simulink model "Codegen"  (Simulink 10.2)
settings: Solver=FixedStepDiscrete  StartTime=0.0  StopTime=10.0  FixedStep=dT  RelTol=1e-3  EnableMultiTasking=on
values from neighbouring files (symbols this model uses):
  a1 = mpt.Parameter    [data_object_def.m]
  a2 = mpt.Parameter    [data_object_def.m]
  b1 = mpt.Parameter    [data_object_def.m]
  b2 = mpt.Parameter    [data_object_def.m]
  dT = mpt.Parameter    [data_object_def.m]
  eta = mpt.Parameter    [data_object_def.m]
  Kp = mpt.Parameter    [data_object_def.m]
  Td = mpt.Parameter    [data_object_def.m]
  Ti = mpt.Parameter    [data_object_def.m]
undefined symbols (not defined in the file or in its folder): DiscIntNeverNeededParam
settings Model: Creator=h-mita  LastModifiedBy=yuto
settings DataIOCC: LimitDataPoints=on
settings OptimizationCC: DefaultParameterBehavior=Inlined  ExpressionDepthLimit=2147483647  InitFltsAndDblsToZero=on  LifeSpan=1  EfficientTunableParamExpr=on
settings DebuggingCC: SolverPrmCheckMsg=warning  StateNameClashWarn=warning
settings SFSimCC: SimUseLocalCustomCode=on  MATLABDynamicMemAlloc=off  CustomCodeUndefinedFunction=FilterOut
settings RTWCC: Description=Real-Time Workshop Embedded Coder (no auto configuration)  SystemTargetFile=ert.tlc  GenCodeOnly=on  TemplateMakefile=ert_default_tmf  RTWUseLocalCustomCode=on
settings CodeAppCC: IgnoreCustomStorageClasses=off  CustomSymbolStrType=$N$R$M  InternalIdentifier=Classic
settings ERTTargetCC: GenerateSampleERTMain=on  IncludeMdlTerminateFcn=off  SupportAbsoluteTime=off  SupportComplex=off  InlinedParameterPlacement=NonHierarchical  ERTCustomFileTemplate=example_file_process.tlc  ConvertIfToSwitch=off  SuppressUnreachableDefaultCases=off
settings ConfigComp: CovExternalEMLEnable=on

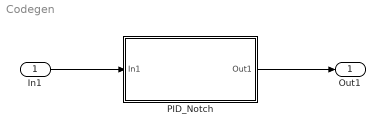
== system Codegen ==
  In1 : Inport
  PID_Notch : Subsystem
  Out1 : Outport  OutDataTypeStr=double
  wires:
  In1/1 -> PID_Notch/1(In1)
  PID_Notch/1(Out1) -> Out1/1

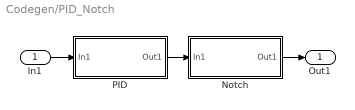
== system Codegen/PID_Notch ==
  In1 : Inport
  Notch : Subsystem
  PID : Subsystem
  Out1 : Outport
  wires:
  PID/1(Out1) -> Notch/1(In1)
  Notch/1(Out1) -> Out1/1
  In1/1 -> PID/1(In1)

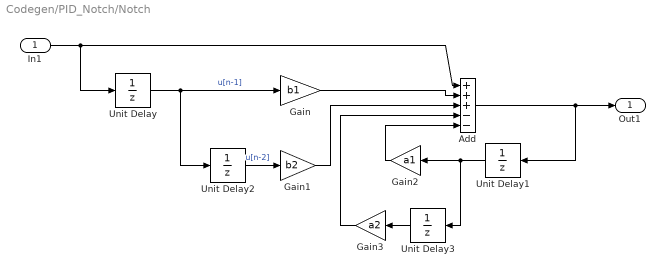
== system Codegen/PID_Notch/Notch ==
  In1 : Inport
  Add : Sum  Inputs=+++--
  Gain : Gain  Gain=b1
  Gain1 : Gain  Gain=b2
  Gain2 : Gain  Gain=a1
  Gain3 : Gain  Gain=a2
  Unit Delay : UnitDelay  SampleTime=-1  StateName=Notch_Unit_Delay  StateMustResolveToSignalObject=on
  Unit Delay1 : UnitDelay  SampleTime=-1  StateName=Notch_Unit_Delay1  StateMustResolveToSignalObject=on
  Unit Delay2 : UnitDelay  SampleTime=-1  StateName=Notch_Unit_Delay2  StateMustResolveToSignalObject=on
  Unit Delay3 : UnitDelay  SampleTime=-1  StateName=Notch_Unit_Delay3  StateMustResolveToSignalObject=on
  Out1 : Outport
  wires:
  Unit Delay/1 -> Gain/1, Unit Delay2/1  "u[n-1]"
  Unit Delay2/1 -> Gain1/1  "u[n-2]"
  Gain1/1 -> Add/3
  Gain/1 -> Add/2
  Add/1 -> Unit Delay1/1, Out1/1
  Unit Delay1/1 -> Gain2/1, Unit Delay3/1
  Gain2/1 -> Add/5
  Unit Delay3/1 -> Gain3/1
  Gain3/1 -> Add/4
  In1/1 -> Unit Delay/1, Add/1

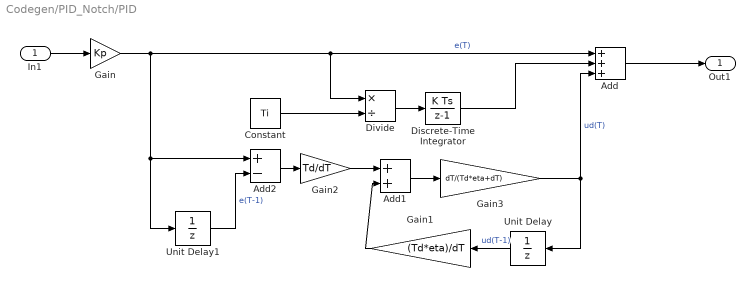
== system Codegen/PID_Notch/PID ==
  In1 : Inport
  Add : Sum  Inputs=+++
  Add1 : Sum
  Add2 : Sum  Inputs=+-
  Constant : Constant  Value=Ti
  Discrete-Time Integrator : DiscreteIntegrator  gainval=1  SampleTime=dT  StateName=PID_Disc_Integrator  ICPrevOutput=DiscIntNeverNeededParam  ICPrevScaledInput=DiscIntNeverNeededParam  StateMustResolveToSignalObject=on
  Divide : Product  Inputs=*/
  Gain : Gain  Gain=Kp
  Gain1 : Gain  Gain=(Td*eta)/dT
  Gain2 : Gain  Gain=Td/dT
  Gain3 : Gain  Gain=dT/(Td*eta+dT)
  Unit Delay : UnitDelay  SampleTime=-1  StateName=PID_Unit_Delay  StateMustResolveToSignalObject=on
  Unit Delay1 : UnitDelay  SampleTime=-1  StateName=PID_Unit_Delay1  StateMustResolveToSignalObject=on
  Out1 : Outport
  wires:
  Gain/1 -> Add/1, Divide/1, Add2/1, Unit Delay1/1  "e(T)"
  Discrete-Time Integrator/1 -> Add/2
  Gain3/1 -> Unit Delay/1, Add/3  "ud(T)"
  Unit Delay/1 -> Gain1/1  "ud(T-1)"
  Gain1/1 -> Add1/2
  Gain2/1 -> Add1/1
  Unit Delay1/1 -> Add2/2  "e(T-1)"
  Add2/1 -> Gain2/1
  Add1/1 -> Gain3/1
  In1/1 -> Gain/1
  Add/1 -> Out1/1
  Divide/1 -> Discrete-Time Integrator/1
  Constant/1 -> Divide/2
